simulink model "fuzzy_pid"  (R2014b)
settings: Solver=ode3  StartTime=0.0  StopTime=4  FixedStep=0.0001  RelTol=1e-3
PreLoadFcn:
  | VarName=readfis('e_ec_u.fis');
libraries: simulink x2, fuzblock x1
settings Model: Creator=JRCHAN  LastModifiedBy=JRCHAN
settings OptimizationCC: BooleanDataType=off

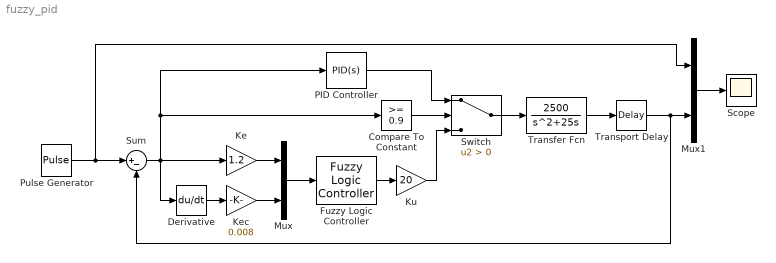
== system fuzzy_pid ==
  Compare To Constant : simulink/Logic and Bit Operations/Compare To Constant  relop=>=  const=0.9  OutDataTypeStr=boolean
  Derivative : Derivative
  Fuzzy Logic Controller : fuzblock/Fuzzy Logic  Controller  fis=[VarName]
  Ke : Gain  Gain=1.2
  Kec : Gain  Gain=0.008
  Ku : Gain  Gain=20
  Mux : Mux  Inputs=2
  Mux1 : Mux  Inputs=2
  PID Controller : simulink/Continuous/PID Controller  Controller=PID  TimeDomain=Continuous-time  SampleTime=-1  IntegratorMethod=Forward Euler  FilterMethod=Forward Euler  Form=Parallel  P=0.3  I=0.05  D=0.01  N=100  InitialConditionSource=internal  InitialConditionForIntegrator=0  InitialConditionForFilter=0  ExternalReset=none  LimitOutput=off  UpperSaturationLimit=inf  LowerSaturationLimit=-inf  LinearizeAsGain=on  AntiWindupMode=none  Kb=1  TrackingMode=off  Kt=1  PParamMin=[]  PParamMax=[]  IParamMin=[]  IParamMax=[]  DParamMin=[]  DParamMax=[]  NParamMin=[]  NParamMax=[]  KbParamMin=[]  KbParamMax=[]  KtParamMin=[]  KtParamMax=[]  POutMin=[]  POutMax=[]  IOutMin=[]  IOutMax=[]  DOutMin=[]  DOutMax=[]  NOutMin=[]  NOutMax=[]  KbOutMin=[]  KbOutMax=[]  KtOutMin=[]  KtOutMax=[]  IntegratorOutMin=[]  IntegratorOutMax=[]  FilterOutMin=[]  FilterOutMax=[]  SumOutMin=[]  SumOutMax=[]  SumI1OutMin=[]  SumI1OutMax=[]  SumI2OutMin=[]  SumI2OutMax=[]  SumI3OutMin=[]  SumI3OutMax=[]  SumDOutMin=[]  SumDOutMax=[]  SaturationOutMin=[]  SaturationOutMax=[]  IntegratorContinuousStateAttributes=''  IntegratorStateMustResolveToSignalObject=off  IntegratorRTWStateStorageClass=Auto  FilterContinuousStateAttributes=''  FilterStateMustResolveToSignalObject=off  FilterRTWStateStorageClass=Auto  DifferentiatorICPrevScaledInput=0  DifferentiatorOutMin=[]  DifferentiatorOutMax=[]  UseFilter=on
  Pulse Generator : DiscretePulseGenerator  PulseType=Time based  Period=1  PulseWidth=50
  Scope : Scope
      settings: TimeRange=5  YMin=-0.4  YMax=2
  Sum : Sum  Inputs=|+-
  Switch : Switch  Criteria=u2 > Threshold
  Transfer Fcn : TransferFcn  Numerator=[2500]  Denominator=[1 25 0]
  Transport Delay : TransportDelay  DelayTime=0.002
  wires:
  Transfer Fcn/1 -> Transport Delay/1
  Pulse Generator/1 -> Mux1/1, Sum/1
  Sum/1 -> Compare To Constant/1, PID Controller/1, Derivative/1, Ke/1
  Derivative/1 -> Kec/1
  Mux/1 -> Fuzzy Logic Controller/1
  Fuzzy Logic Controller/1 -> Ku/1
  Transport Delay/1 -> Sum/2, Mux1/2
  Mux1/1 -> Scope/1
  Ke/1 -> Mux/1
  Kec/1 -> Mux/2
  Ku/1 -> Switch/3
  Compare To Constant/1 -> Switch/2
  PID Controller/1 -> Switch/1
  Switch/1 -> Transfer Fcn/1
